simulink model "VehCtrlMdel240829_2018b"  (R2019b)
settings: Solver=FixedStepDiscrete  StartTime=0.0  StopTime=10.0  FixedStep=0.0005  RelTol=1e-3  EnableMultiTasking=on
values from neighbouring files (symbols this model uses):
  Ax_OffSet = 0.0    [VehCtrlMdelDictionary.sldd]
  Ay_OffSet = 0.0    [VehCtrlMdelDictionary.sldd]
  Caf = 460.0    [VehCtrlMdelDictionary.sldd]    (also in trqvparameter.m = 460)
  Car = 440.0    [VehCtrlMdelDictionary.sldd]    (also in trqvparameter.m = 440)
  dwf = 1.2    [VehCtrlMdelDictionary.sldd]    (also in trqvparameter.m)
  Iz = 105.0    [VehCtrlMdelDictionary.sldd]    (also in trqvparameter.m = 105)
  Ki = 1.0    [VehCtrlMdelDictionary.sldd]    (also in trqvparameter.m = 20)
  Kp = 2.0    [VehCtrlMdelDictionary.sldd]    (also in trqvparameter.m = 30)
  Ldwf = 1.2    [VehCtrlMdelDictionary.sldd]    (also in trqvparameter.m)
  Ldwr = 1.16    [VehCtrlMdelDictionary.sldd]    (also in trqvparameter.m)
  lf = 0.761    [VehCtrlMdelDictionary.sldd]    (also in trqvparameter.m)
  lr = 0.831    [VehCtrlMdelDictionary.sldd]    (also in trqvparameter.m)
  m = 340.0    [VehCtrlMdelDictionary.sldd]    (also in trqvparameter.m = 340)
  Offset_Angle = 0.0    [VehCtrlMdelDictionary.sldd]
  Qa = 0.1    [VehCtrlMdelDictionary.sldd]    (also in trqvparameter.m)
  Ra = 2.0    [VehCtrlMdelDictionary.sldd]    (also in trqvparameter.m = 2)
  RearRatio = 0.8    [VehCtrlMdelDictionary.sldd]
  Rt = 0.2    [VehCtrlMdelDictionary.sldd]    (also in trqvparameter.m)
  thr1 = 2.0    [VehCtrlMdelDictionary.sldd]    (also in trqvparameter.m = 2)
  thr2 = 0.5    [VehCtrlMdelDictionary.sldd]    (also in trqvparameter.m)
  thr3 = 0.8    [VehCtrlMdelDictionary.sldd]    (also in trqvparameter.m)
  thr4 = 0.5    [VehCtrlMdelDictionary.sldd]    (also in trqvparameter.m)
  thr5 = -0.5    [VehCtrlMdelDictionary.sldd]    (also in trqvparameter.m)
  TrqRquRate = 0.1    [VehCtrlMdelDictionary.sldd]    (also in trqvparameter.m)
  YawRate_OffSet = 0.0    [VehCtrlMdelDictionary.sldd]
undefined symbols (not defined in the file or in its folder): DiscIntNeverNeededParam, I_AN07_5V, I_AN08_5V, I_AN10_5V, I_SW01_L, I_SW02_L, I_SW03_L, O_SW12_HS1A, O_SW14_HS1A, PWM3
libraries: simulink x126, ec5744lib x77, canmsglib x18
(part 2 of 5)

== system VehCtrlMdel240829_2018b/OUTPUT/VCU2CLUSTER ==
  In1 : Inport
  TCS : Inport  Port=2
  function : TriggerPort  TriggerType=function-call  VariantControl=Variant
  Bus Selector : BusSelector  OutputSignals=signal2.APPBrk_BUS.Brk_F,signal2.MCU.MCU_state.Trq,signal2.APPBrk_BUS.Acc_POS,signal2.MCU.MCU_pwr.motor_temp,signal2.VehSpd_FLkph,signal2.MCU.MCU_state.Spd_R_kph,signal2.APPBrk_BUS.Brk_R,signal2.MCU.MCU_state.RPM
  Bus Selector1 : BusSelector  OutputSignals=TCS_TrqRequestFinal_Nm,TCS_flgActv
  CAN Pack : canmsglib/CAN Pack  CANdbFile=E:\candbc\cluster.dbc  MsgList=(none)  MsgName=New_Message_1  MsgIDType=Standard (11-bit identifier)  MsgIdentifier=291  MsgLength=8  Remote=off  ApplyMinMax=off  BusOutput=off  SignalInfo={'Brk_F','56','8','LE','signed','Standard','0','30','100','-3740','3910';'TCS_Trq_cmd','40','8','LE','unsigned','Standard','0','1','0','0','255';'TCS_flag','32','8','LE','signed','Standard','0','1','0','-Inf','Inf';'Trq_feedback','48','8','LE','signed','Standard','0','1','0','-128','250';'acc','24','8','LE','unsigned','Standard','0','1','0','0','100';'motor_temp','0','8','LE','unsigned','Standard','0','1','0','0','100';'veh_spd_F','8','8','LE','unsigned','Standard','0','1','0','0','120';'veh_spd_R','16','8','LE','unsigned','Standard','0','1','0','0','120'}
      settings: SourceProductName=Vehicle Network Toolbox  SourceProductBaseCode=VN  DataFormat=CANdb specified signals
  CAN Pack1 : canmsglib/CAN Pack  CANdbFile=E:\candbc\cluster.dbc  MsgList=(none)  MsgName=New_Message_2  MsgIDType=Standard (11-bit identifier)  MsgIdentifier=292  MsgLength=2  Remote=off  ApplyMinMax=off  BusOutput=off  SignalInfo={'Brk_R','0','8','LE','signed','Standard','0','30','100','-Inf','Inf';'RPM_feedback','8','8','LE','signed','Standard','0','1','0','-Inf','Inf'}
      settings: SourceProductName=Simulink Real-Time  SourceProductBaseCode=XP  DataFormat=CANdb specified signals
  CANPackMessage : ec5744lib/RapidECU_U3/04CANCommunication/CANPackMessage  datalength=8  sampletime=-1
      settings: SourceProductName=ECUCoder for MPC5744
  CANPackMessage1 : ec5744lib/HYFCU001/04CANCommunication/CANPackMessage  datalength=8  sampletime=-1
      settings: SourceProductName=ECUCoder for MPC5744
  CANTransmit : ec5744lib/RapidECU_U3/04CANCommunication/CANTransmit  canmodule=0  canbuffer=9  canmessageid=291  canmessagetype=Standard(11-bit ID)  datalength=8  sampletime=-1
      settings: SourceProductName=ECUCoder for MPC5744
  CANTransmit1 : ec5744lib/RapidECU_U3/04CANCommunication/CANTransmit  canmodule=0  canbuffer=10  canmessageid=292  canmessagetype=Standard(11-bit ID)  datalength=8  sampletime=-1
      settings: SourceProductName=ECUCoder for MPC5744
  Terminator1 : Terminator
  Terminator3 : Terminator
  wires:
  CANTransmit/1 -> Terminator3/1
  CANPackMessage/1 -> CANTransmit/1
  CAN Pack/1 -> CANPackMessage/1
  In1/1 -> Bus Selector/1
  Bus Selector/5 -> CAN Pack/7  "<VehSpd_FLkph>"
  Bus Selector/4 -> CAN Pack/6  "<motor_temp>"
  Bus Selector/3 -> CAN Pack/5  "<Acc_POS>"
  Bus Selector/6 -> CAN Pack/8  "<Spd_R_kph>"
  Bus Selector/1 -> CAN Pack/1  "<Brk_F>"
  Bus Selector/2 -> CAN Pack/4  "<Trq>"
  TCS/1 -> Bus Selector1/1
  Bus Selector1/2 -> CAN Pack/3  "<TCS_flgActv>"
  Bus Selector1/1 -> CAN Pack/2  "<TCS_TrqRequestFinal_Nm>"
  Bus Selector/7 -> CAN Pack1/1  "<Brk_R>"
  Bus Selector/8 -> CAN Pack1/2  "<RPM>"
  CAN Pack1/1 -> CANPackMessage1/1
  CANPackMessage1/1 -> CANTransmit1/1
  CANTransmit1/1 -> Terminator1/1

== system VehCtrlMdel240829_2018b/OUTPUT/VCU2EmraxMCU ==
  note: 0: 0Nm
      | 2: Trq mode
  note: 0: N
      | 2:D
  note: 加ramp
  note: 1.spd改成motor_rpm
      | 2.APP_bad改成acc_error
      | 3.设置模式的优先级
      | 4.车轮低负载（悬空），加最高车速限制
  In1 : Inport
  function : TriggerPort  TriggerType=function-call  VariantControl=(inherit)
  Bus Selector : BusSelector  OutputSignals=Trq_CUT,TrqR_cmd,VCU_SpdCmd_Emrax
  CAN Pack1 : canmsglib/CAN Pack  CANdbFile=E:\candbc\MCU_No1.dbc  MsgList=(none)  MsgName=VCU2MCU1_ID1  MsgIDType=Extended (29-bit identifier)  MsgIdentifier=146927393  MsgLength=8  Remote=off  ApplyMinMax=off  BusOutput=off  SignalInfo={'VCU2MCU_Control_mode_ID1','32','8','LE','unsigned','Standard','0','1','0','0','255';'VCU2MCU_Gear_ID1','40','2','LE','unsigned','Standard','0','1','0','0','3';'VCU2MCU_Speed_Limit_ID1','0','16','LE','unsigned','Standard','0','5.000000e-01','-10000','-10000','10000';'VCU2MCU_Torque_Control_ID1','16','16','LE','unsigned','Standard','0','1','0','0','1000'}
      settings: SourceProductName=Vehicle Network Toolbox  SourceProductBaseCode=VN  DataFormat=CANdb specified signals
  CANPackMessage : ec5744lib/RapidECU_U3/04CANCommunication/CANPackMessage  datalength=8  sampletime=-1
      settings: SourceProductName=ECUCoder for MPC5744
  CANTransmit : ec5744lib/RapidECU_U3/04CANCommunication/CANTransmit  canmodule=0  canbuffer=8  canmessageid=146927393  canmessagetype=Extended(29-bit ID)  datalength=8  sampletime=-1
      settings: SourceProductName=ECUCoder for MPC5744
  Cast To Boolean4 : DataTypeConversion  OutDataTypeStr=uint16
  Cast To Boolean6 : DataTypeConversion  OutDataTypeStr=uint16
  Constant13 : Constant  Value=2
  Constant17 : Constant  Value=0
  Constant19 : Constant  Value=2
  Constant20 : Constant  Value=0
  Data Type Conversion1 : DataTypeConversion  OutDataTypeStr=single
  Data Type Conversion2 : DataTypeConversion  OutDataTypeStr=int32
  MeaModule1 : ec5744lib/HYFCU001/07Calibration/MeaModule  signal=Gear_Trs
      settings: SourceProductName=ECUCoder for MPC5744
  MeaModule2 : ec5744lib/HYFCU001/07Calibration/MeaModule  signal=Mode_Trs
      settings: SourceProductName=ECUCoder for MPC5744
  Ramp : simulink/Sources/Ramp  Commented=on  slope=1  start=0  InitialOutput=0
  Switch2 : Switch  Criteria=u2 > Threshold
  Switch3 : Switch  Criteria=u2 > Threshold
  Terminator3 : Terminator
  wires:
  CANTransmit/1 -> Terminator3/1
  CAN Pack1/1 -> CANPackMessage/1
  CANPackMessage/1 -> CANTransmit/1
  MeaModule1/1 -> Cast To Boolean4/1
  Bus Selector/2 -> Data Type Conversion1/1  "<TrqR_cmd>"
  Constant20/1 -> Switch2/1
  Bus Selector/1 -> Switch2/2, Switch3/2  "<Trq_CUT>"
  Constant19/1 -> Switch2/3
  Constant13/1 -> Switch3/3
  Constant17/1 -> Switch3/1
  Switch3/1 -> MeaModule2/1
  Switch2/1 -> MeaModule1/1
  MeaModule2/1 -> Cast To Boolean6/1
  Data Type Conversion1/1 -> CAN Pack1/3
  Data Type Conversion2/1 -> CAN Pack1/4
  Cast To Boolean4/1 -> CAN Pack1/1
  Cast To Boolean6/1 -> CAN Pack1/2
  Bus Selector/3 -> Data Type Conversion2/1  "<VCU_SpdCmd_Emrax>"
  In1/1 -> Bus Selector/1

== system VehCtrlMdel240829_2018b/OUTPUT/WP_OUTPUT ==
  note: 数据类型转换
  aWaterPumpON : Inport
  LoadOfbWaterPump : Inport  Port=2
  function : TriggerPort  TriggerType=function-call  VariantControl=(inherit)
  Cast To Single : DataTypeConversion  OutDataTypeStr=boolean
  Cast To Single1 : DataTypeConversion  OutDataTypeStr=uint16
  Constant : Constant  Value=uint16(1000)  OutDataTypeStr=uint16  SampleTime=-1
  PowerDriverPWM : ec5744lib/RapidECU_U3/03PowerDriverPWM/PowerDriverPWM  channel=114:O_SW12_HS1A/PWM3  sampletime=-1
      settings: SourceProductName=ECUCoder for MPC5744
  PowerDriverSwitch(HS) : ec5744lib/RapidECU_U3/02PowerDriverSwitch/PowerDriverSwitch(HS)  channel=114:O_SW12_HS1A  sampletime=-1
      settings: SourceProductName=ECUCoder for MPC5744
  wires:
  LoadOfbWaterPump/1 -> Cast To Single1/1
  Constant/1 -> PowerDriverPWM/1
  aWaterPumpON/1 -> Cast To Single/1
  Cast To Single/1 -> PowerDriverSwitch(HS)/1
  Cast To Single1/1 -> PowerDriverPWM/2

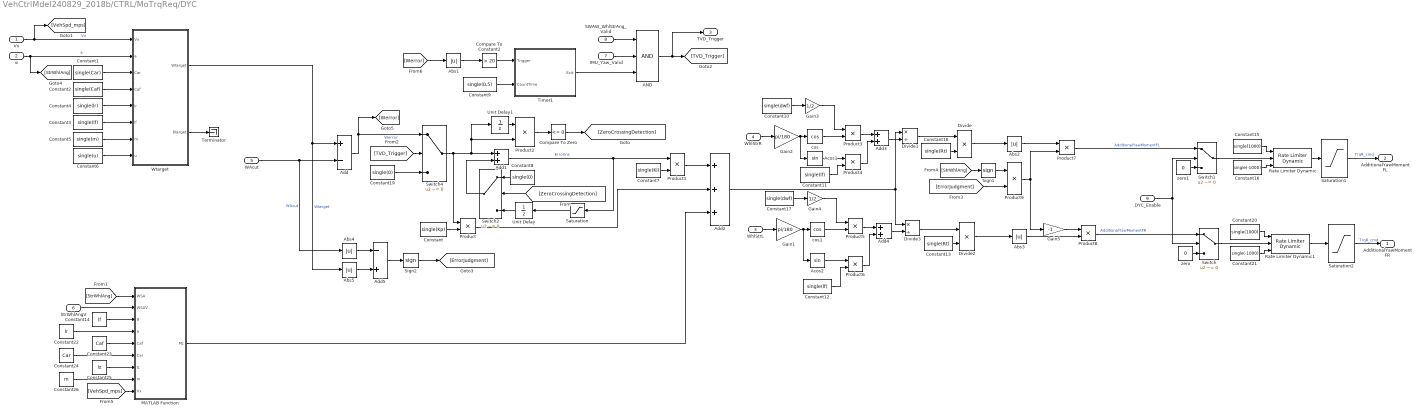
== system VehCtrlMdel240829_2018b/CTRL/MoTrqReq/DYC ==
  Vx : Inport
  α : Inport  Port=2
  WhlStrL : Inport  Port=3
  WhlStrR : Inport  Port=4
  WAcut : Inport  Port=5
  StrWhlAngV : Inport  Port=6
  IMU_Yaw_Valid : Inport  Port=7
  SWAW_WhlStrAng_Valid : Inport  Port=8
  "DYC_Enable " : Inport  Port=9
  AND : Logic  Inputs=3  AllPortsSameDT=off  OutDataTypeStr=boolean
  Abs{1..5} (5 alike) : Abs
  Acos1 : Trigonometry
  Acos2 : Trigonometry
  Add : Sum  Inputs=+-
  Add1 : Sum
  Add2 : Sum  Inputs=+++
  Add3 : Sum
  Add4 : Sum
  Add5 : Sum  Inputs=-+
  Compare To Constant2 : simulink/Logic and Bit Operations/Compare To Constant  relop=>  const=20  OutDataTypeStr=boolean
  Compare To Zero : simulink/Logic and Bit Operations/Compare To Zero  relop=<=  OutDataTypeStr=boolean
  Constant : Constant  Value=single(Kp)
  Constant1 : Constant  Value=single(Car)
  Constant10 : Constant  Value=single(dwf)
  Constant11 : Constant  Value=single(lf)
  Constant12 : Constant  Value=single(lf)
  Constant13 : Constant  Value=single(Rt)
  Constant14 : Constant  Value=lf
  Constant15 : Constant  Value=single(1000)
  Constant16 : Constant  Value=single(-1000)
  Constant17 : Constant  Value=single(dwf)
  Constant18 : Constant  Value=single(Rt)
  Constant19 : Constant  Value=single(0)
  Constant2 : Constant  Value=single(Caf)
  Constant20 : Constant  Value=single(1000)
  Constant21 : Constant  Value=single(-1000)
  Constant22 : Constant  Value=lr
  Constant23 : Constant  Value=Caf
  Constant24 : Constant  Value=Car
  Constant25 : Constant  Value=Iz
  Constant26 : Constant  Value=m
  Constant3 : Constant  Value=single(lf)
  Constant4 : Constant  Value=single(lr)
  Constant5 : Constant  Value=single(m)
  Constant6 : Constant  Value=single(u)
  Constant7 : Constant  Value=single(Ki)
  Constant8 : Constant  Value=single(0)
  Constant9 : Constant  Value=single(0.5)
  Divide : Product  Inputs=**
  Divide1 : Product  Inputs=*/
  Divide2 : Product  Inputs=**
  Divide3 : Product  Inputs=*/
  Gain1 : Gain  Gain=pi/180
  Gain2 : Gain  Gain=pi/180
  Gain3 : Gain  Gain=1/2
  Gain4 : Gain  Gain=1/2
  Gain5 : Gain  Gain=-1
  MATLAB Function : MATLAB Function  TreatAsAtomicUnit=on
  Product{,1..9} (10 alike) : Product
  Rate Limiter Dynamic : simulink/Discontinuities/Rate Limiter Dynamic
      settings: SourceProductName=Simulink
  Rate Limiter Dynamic1 : simulink/Discontinuities/Rate Limiter Dynamic
      settings: SourceProductName=Simulink
  Saturation : Saturate  UpperLimit=10  LowerLimit=-10
  Saturation1 : Saturate  UpperLimit=20  LowerLimit=-20
  Saturation2 : Saturate  UpperLimit=20  LowerLimit=-20
  Sign1 : Signum
  Sign2 : Signum
  Switch{,1..2,4} (4 alike) : Switch  Criteria=u2 ~= 0
  Terminator : Terminator
  Timer1 : Stateflow chart  TreatAsAtomicUnit=on
  Unit Delay : UnitDelay  SampleTime=-1  HasFrameUpgradeWarning=on
  Unit Delay1 : UnitDelay  SampleTime=-1  HasFrameUpgradeWarning=on
  Wtarget : MATLAB Function  TreatAsAtomicUnit=on
  cos : Trigonometry  Operator=cos
  cos1 : Trigonometry  Operator=cos
  zero : Constant  Value=0
  zero1 : Constant  Value=0
  AdditionalYawMomentFR : Outport  VectorParamsAs1DForOutWhenUnconnected=off
  AdditionalYawMomentFL : Outport  Port=2  VectorParamsAs1DForOutWhenUnconnected=off
  TVD_Trigger : Outport  Port=3  VectorParamsAs1DForOutWhenUnconnected=off
  wires:
  Constant2/1 -> Wtarget/4(Caf)
  Wtarget/1(Wtarget) -> Add/1, Abs5/1  "Wtarget"
  Vx/1 -> [VehSpd_mps], Wtarget/1(Vx)  "Vx"
  Constant6/1 -> Wtarget/8(u)
  Constant5/1 -> Wtarget/7(m)
  Constant1/1 -> Wtarget/3(Car)
  Constant3/1 -> Wtarget/6(lf)
  α/1 -> [StrWhlAng], Wtarget/2(a)  "a"
  Constant4/1 -> Wtarget/5(lr)
  Product8/1 -> Switch/1  "AdditionalYawMomentFR"
  Product7/1 -> Switch1/1  "AdditionalYawMomentFL"
  Wtarget/2(btarget) -> Terminator/1
  Switch/1 -> Rate Limiter Dynamic1/2
  Switch1/1 -> Rate Limiter Dynamic/2
  "DYC_Enable "/1 -> Switch1/2, Switch/2
  zero/1 -> Switch/3
  zero1/1 -> Switch1/3
  Compare To Zero/1 -> [ZeroCrossingDetection]
  Abs3/1 -> Product8/2
  Abs5/1 -> Add5/2
  Abs4/1 -> Add5/1
  Constant19/1 -> Switch4/3
  Add5/1 -> Sign2/1
  Constant12/1 -> Product6/2
  Sign2/1 -> [ErrorJudgment]
  Saturation/1 -> Unit Delay/1
  Divide/1 -> Abs2/1
  [ErrorJudgment] -> Product9/2
  Unit Delay/1 -> Switch2/3
  Add1/1 -> Saturation/1, Product1/1  "ErrorIns"
  Add3/1 -> Divide1/2
  Gain5/1 -> Product8/1
  Product4/1 -> Add3/2
  Abs2/1 -> Product7/1
  Acos2/1 -> Product6/1
  Add/1 -> [Werror], Switch4/1  "Werror"
  Gain1/1 -> cos1/1, Acos2/1
  Constant15/1 -> Rate Limiter Dynamic/1
  Divide1/1 -> Divide/1
  WhlStrL/1 -> Gain1/1
  cos/1 -> Product3/2
  [TVD_Trigger] -> Switch4/2
  Constant11/1 -> Product4/2
  Product5/1 -> Add4/1
  Product3/1 -> Add3/1
  Constant10/1 -> Gain3/1
  Gain2/1 -> Acos1/1, cos/1
  Gain3/1 -> Product3/1
  Constant8/1 -> Switch2/1
  Product6/1 -> Add4/2
  Acos1/1 -> Product4/1
  WhlStrR/1 -> Gain2/1
  Add4/1 -> Divide3/2
  Constant18/1 -> Divide/2
  Constant17/1 -> Gain4/1
  Switch4/1 -> Add1/1, Unit Delay1/1, Product2/2, Product/1
  WAcut/1 -> Add/2, Abs4/1  "WAcut"
  Product/1 -> Add2/2
  Abs1/1 -> Compare To Constant2/1
  [ZeroCrossingDetection] -> Switch2/2
  Compare To Constant2/1 -> Timer1/1(Trigger)
  Divide3/1 -> Divide2/1
  Gain4/1 -> Product5/1
  Constant13/1 -> Divide2/2
  Switch2/1 -> Add1/2
  Product9/1 -> Gain5/1, Product7/2
  cos1/1 -> Product5/2
  Constant16/1 -> Rate Limiter Dynamic/3
  Sign1/1 -> Product9/1
  Divide2/1 -> Abs3/1
  Constant/1 -> Product/2
  Constant7/1 -> Product1/2
  Product1/1 -> Add2/1
  Rate Limiter Dynamic/1 -> Saturation1/1
  Constant21/1 -> Rate Limiter Dynamic1/3
  Constant20/1 -> Rate Limiter Dynamic1/1
  Rate Limiter Dynamic1/1 -> Saturation2/1
  Add2/1 -> Divide3/1, Divide1/1
  Saturation1/1 -> AdditionalYawMomentFL/1  "TrqR_cmd"
  Saturation2/1 -> AdditionalYawMomentFR/1  "TrqR_cmd"
  [StrWhlAng] -> Sign1/1
  StrWhlAngV/1 -> MATLAB Function/2(WSAV)
  Constant9/1 -> Timer1/2(CountTime)
  Timer1/1(Exit) -> AND/3
  IMU_Yaw_Valid/1 -> AND/2
  SWAW_WhlStrAng_Valid/1 -> AND/1
  AND/1 -> TVD_Trigger/1, [TVD_Trigger]
  MATLAB Function/1(Mz) -> Add2/3
  [StrWhlAng] -> MATLAB Function/1(WSA)
  Constant14/1 -> MATLAB Function/3(lf)
  Constant22/1 -> MATLAB Function/4(lr)
  Constant23/1 -> MATLAB Function/5(Caf)
  Constant24/1 -> MATLAB Function/6(Car)
  Constant25/1 -> MATLAB Function/7(Iz)
  Constant26/1 -> MATLAB Function/8(m)
  [VehSpd_mps] -> MATLAB Function/9(Vx)
  Unit Delay1/1 -> Product2/1
  Product2/1 -> Compare To Zero/1
  [Werror] -> Abs1/1

== system VehCtrlMdel240829_2018b/CTRL/MoTrqReq/Subsystem ==
  SingleAMKPowerLimit_KW : Inport
  SingleEmraxPowerLimit_KW : Inport  Port=2
  MCFL_ActualVelocity : Inport  Port=3
  MCFR_ActualVelocity : Inport  Port=4
  RPM : Inport  Port=5
  Add : Sum  Inputs=+-
  Add1 : Sum
  Add2 : Sum
  Add3 : Sum
  Add4 : Sum  Inputs=+-
  Constant : Constant
  Constant1 : Constant  Value=single(9550)  OutDataTypeStr=single
  Constant2 : Constant  Value=single(9550)  OutDataTypeStr=single
  Constant3 : Constant
  Constant5 : Constant  Value=single(9550)  OutDataTypeStr=single
  Divide : Product  Inputs=*/
  Divide1 : Product  Inputs=*/
  Divide2 : Product  Inputs=*/
  Max : MinMax  Function=max  Inputs=2
  Max1 : MinMax  Function=max  Inputs=2
  Max2 : MinMax  Function=max  Inputs=2
  MaxPwr : Constant  Value=single(63)  OutDataTypeStr=single
  MaxPwr1 : Constant  Value=single(7)  OutDataTypeStr=single
  MaxPwr2 : Constant  Value=single(7)  OutDataTypeStr=single
  Product{,1..5} (6 alike) : Product
  RPM_min : Constant  Value=single(10)  OutDataTypeStr=single
  RPM_min1 : Constant  Value=single(1)  OutDataTypeStr=single
  RPM_min2 : Constant  Value=single(10)  OutDataTypeStr=single
  RPM_min3 : Constant  Value=single(1)  OutDataTypeStr=single
  RPM_min4 : Constant  Value=single(10)  OutDataTypeStr=single
  RPM_min5 : Constant  Value=single(1)  OutDataTypeStr=single
  TrqLimEmrax_Nm : Outport
  TrqLimFR_Nm : Outport  Port=2
  TrqLimFL_Nm : Outport  Port=3
  wires:
  Max/1 -> Divide/2
  Divide/1 -> TrqLimEmrax_Nm/1  "TrqLim_Nm"
  RPM_min1/1 -> Max/2
  Constant5/1 -> Product/2
  RPM/1 -> Add1/1
  Product/1 -> Divide/1
  RPM_min/1 -> Add1/2
  Add1/1 -> Max/1
  Add2/1 -> Max1/1
  RPM_min2/1 -> Add2/2
  MaxPwr1/1 -> Product4/1
  Product1/1 -> Divide1/1
  MCFR_ActualVelocity/1 -> Add2/1
  Constant1/1 -> Product1/2
  RPM_min3/1 -> Max1/2
  Divide1/1 -> TrqLimFR_Nm/1  "TrqLim_Nm"
  Max1/1 -> Divide1/2
  Max2/1 -> Divide2/2
  Divide2/1 -> TrqLimFL_Nm/1  "TrqLim_Nm"
  RPM_min5/1 -> Max2/2
  Constant2/1 -> Product2/2
  MCFL_ActualVelocity/1 -> Add3/1
  Product2/1 -> Divide2/1
  RPM_min4/1 -> Add3/2
  Add3/1 -> Max2/1
  MaxPwr/1 -> Product5/1
  Add/1 -> Product5/2
  Product5/1 -> Product/1
  Product3/1 -> Product2/1
  Add4/1 -> Product3/2, Product4/2
  Product4/1 -> Product1/1
  Constant/1 -> Add4/1
  MaxPwr2/1 -> Product3/1
  SingleAMKPowerLimit_KW/1 -> Add4/2
  SingleEmraxPowerLimit_KW/1 -> Add/2
  Constant3/1 -> Add/1

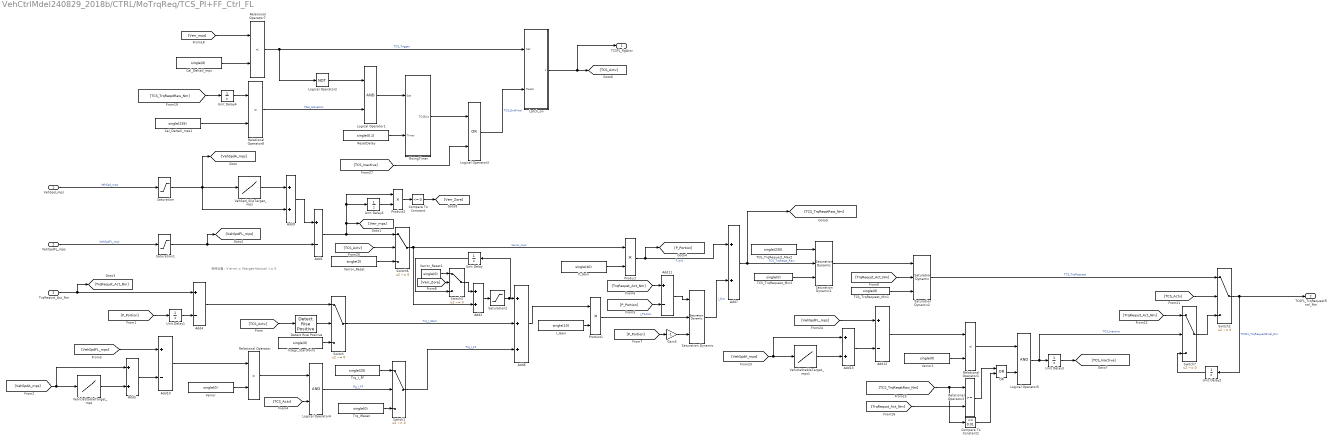
== system VehCtrlMdel240829_2018b/CTRL/MoTrqReq/TCS_PI+FF_Ctrl_FL ==
  note: 特殊设置：V error = Vtarget-Vactual <= 0
  VehSpd_mps : Inport
  VehSpdFL_mps : Inport  Port=2
  TrqRequst_Act_Nm : Inport  Port=3
  Add{1,4,10..12} (5 alike) : Sum  Inputs=+-
  Add{2,5,7,9,13} (5 alike) : Sum
  Add6 : Sum  Inputs=+++
  Cal_DeltaV_mps : Constant  Value=single(0)
  Cal_DeltaV_mps1 : Constant  Value=single(235)
  Compare To Constant : simulink/Logic and Bit Operations/Compare To Constant  relop=<=  const=0  OutDataTypeStr=boolean
  Compare To Constant2 : simulink/Logic and Bit Operations/Compare To Constant  relop=<=  const=0.01  OutDataTypeStr=boolean
  Detect Rise Positive : simulink/Logic and Bit Operations/Detect Rise Positive  vinit=0  OutDataTypeStr=boolean
  Gain3 : Gain  Gain=-1
  I_Gain : Constant  Value=single(10)
  Integr_StartPoint : Constant  Value=single(0)
  Latch_on : Subsystem
  Logical Operator1 : Logic  AllPortsSameDT=off  OutDataTypeStr=boolean
  Logical Operator2 : Logic  Operator=NOT  AllPortsSameDT=off  OutDataTypeStr=boolean
  Logical Operator3 : Logic  Operator=OR  AllPortsSameDT=off  OutDataTypeStr=boolean
  Logical Operator4 : Logic  AllPortsSameDT=off  OutDataTypeStr=boolean
  Logical Operator5 : Logic  AllPortsSameDT=off  OutDataTypeStr=boolean
  OR : Logic  Operator=OR  AllPortsSameDT=off  OutDataTypeStr=boolean
  P_Gain : Constant  Value=single(40)
  Product : Product
  Product1 : Product
  Product2 : Product
  Relational Operator : RelationalOperator  Operator=<  OutDataTypeStr=boolean  RndMeth=Simplest
  Relational Operator1 : RelationalOperator  Operator=<  OutDataTypeStr=boolean  RndMeth=Simplest
  Relational Operator2 : RelationalOperator  OutDataTypeStr=boolean  RndMeth=Simplest
  Relational Operator7 : RelationalOperator  Operator=<  OutDataTypeStr=boolean  RndMeth=Simplest
  Relational Operator8 : RelationalOperator  Operator=>  OutDataTypeStr=boolean  RndMeth=Simplest
  ResetDelay : Constant  Value=single(0.1)
  RisingTimer : Subsystem
  Saturation : Saturate  UpperLimit=40  LowerLimit=0
  Saturation Dynamic : simulink/Discontinuities/Saturation Dynamic  OutMin=[]  OutMax=[]  OutDataTypeStr=Inherit: Same as second input  OutDataType=fixdt(1, 16)  OutScaling=2^-10  DoSatur=off
  Saturation Dynamic1 : simulink/Discontinuities/Saturation Dynamic  OutMin=[]  OutMax=[]  OutDataTypeStr=Inherit: Same as second input  OutDataType=fixdt(1, 16)  OutScaling=2^-10  DoSatur=off
  Saturation Dynamic2 : simulink/Discontinuities/Saturation Dynamic  OutMin=[]  OutMax=[]  OutDataTypeStr=Inherit: Same as second input  OutDataType=fixdt(1, 16)  OutScaling=2^-10  DoSatur=off
  Saturation1 : Saturate  UpperLimit=50  LowerLimit=0
  Saturation2 : Saturate  UpperLimit=400  LowerLimit=-100
  Switch{,1..3,6..7} (6 alike) : Switch  Criteria=u2 ~= 0
  TCS_TrqRequest_Max2 : Constant  Value=single(235)
  TCS_TrqRequest_Min1 : Constant  Value=single(0)
  TCS_TrqRequest_Min2 : Constant  Value=single(0)
  Trq_IReset : Constant  Value=single(0)
  Trq_I_FF : Constant  Value=single(20)
  Unit Delay{,1..5} (6 alike) : UnitDelay  SampleTime=-1  HasFrameUpgradeWarning=on
  VehSpd_SlipTarget_mps : Lookup_n-D  NumberOfTableDimensions=1  BreakpointsForDimension1=[0,3,25,30]  Table=[0.3,0.3,2.5,2.5]  ExtrapMethod=Clip  InternalRulePriority=Speed  RndMeth=Simplest  InputSameDT=on
  VehicleStableTarget_mps : Lookup_n-D  NumberOfTableDimensions=1  BreakpointsForDimension1=[0,3,25,30]  Table=[0.4,0.4,1.2,1.2]  ExtrapMethod=Clip  InternalRulePriority=Speed  RndMeth=Simplest  InputSameDT=on
  VehicleStableTarget_mps1 : Lookup_n-D  NumberOfTableDimensions=1  BreakpointsForDimension1=[0,3,25,30]  Table=[0.4,0.4,1.2,1.2]  ExtrapMethod=Clip  InternalRulePriority=Speed  RndMeth=Simplest  InputSameDT=on
  Verror : Constant  Value=single(0)
  Verror1 : Constant  Value=single(0)
  Verror_Reset : Constant  Value=single(0)
  Verror_Reset1 : Constant  Value=single(0)
  TCSFL_flgActv : Outport
  TCSFL_TrqRequestFinal_Nm : Outport  Port=2
  wires:
  Switch2/1 -> TCSFL_TrqRequestFinal_Nm/1, Unit Delay2/1  "TCSFL_TrqRequestFinal_Nm"
  Saturation/1 -> Add9/2, VehSpd_SlipTarget_mps/1, [VehSpdA_mps]
  Gain3/1 -> Saturation Dynamic/3
  [P_Portion] -> Gain3/1
  P_Gain/1 -> Product/2
  Unit Delay/1 -> Switch3/3
  Add2/1 -> Saturation2/1
  [TrqRequst_Act_Nm] -> Add11/1
  Saturation2/1 -> Unit Delay/1, Add6/1
  Switch/1 -> Add6/2  "Trq_I_Start"
  Saturation Dynamic/1 -> Add7/2  "I_Out"
  VehSpd_mps/1 -> Saturation/1  "VehSpd_mps"
  Saturation1/1 -> Add1/2, [VehSpdFL_mps]
  Product1/1 -> Saturation Dynamic/2  "I_Portion"
  TrqRequst_Act_Nm/1 -> Add4/1, [TrqRequst_Act_Nm]
  Add6/1 -> Product1/1
  TCS_TrqRequest_Min1/1 -> Saturation Dynamic2/3
  Detect Rise Positive/1 -> Switch/2
  Integr_StartPoint/1 -> Switch/3
  I_Gain/1 -> Product1/2
  Saturation Dynamic2/1 -> Switch2/1  "TCS_TrqRequest"
  Add7/1 -> Saturation Dynamic1/2, [TCS_TrqReqstRaw_Nm]  "TCS_TrqReqst_Raw"
  [TrqRequst_Act_Nm] -> Saturation Dynamic2/2
  VehSpd_SlipTarget_mps/1 -> Add9/1
  Add9/1 -> Add1/1
  [Verr_mps] -> Relational Operator7/1
  Cal_DeltaV_mps/1 -> Relational Operator7/2
  Relational Operator7/1 -> Latch_on/1(Set), Logical Operator2/1  "TCS_Trigger"
  [TCS_TrqReqstRaw_Nm] -> Unit Delay4/1
  Logical Operator2/1 -> Logical Operator1/1
  Relational Operator8/1 -> Logical Operator1/2  "fSat_Actuators"
  Cal_DeltaV_mps1/1 -> Relational Operator8/2
  Logical Operator1/1 -> RisingTimer/1(Set)
  ResetDelay/1 -> RisingTimer/2(Timer)
  RisingTimer/1(TCSExit) -> Logical Operator3/1
  Logical Operator3/1 -> Latch_on/2(Reset)  "TCS_ExitFinal"
  Latch_on/1(flg_TCSActv) -> TCSFL_flgActv/1, [TCS_Actv]
  [TCS_Actv] -> Switch6/2
  Verror_Reset/1 -> Switch6/3
  Switch6/1 -> Product/1, Add2/2  "Verror_mps"
  Product/1 -> [P_Portion], Add7/1  "P_out"
  [TCS_Actv] -> Detect Rise Positive/1
  [P_Portion] -> Unit Delay1/1
  Add4/1 -> Switch/1
  Unit Delay1/1 -> Add4/2
  [VehSpdA_mps] -> Add5/1, VehicleStableTarget_mps/1
  VehicleStableTarget_mps/1 -> Add5/2
  Add5/1 -> Add10/2
  [VehSpdFL_mps] -> Add10/1
  Add10/1 -> Relational Operator/1
  Verror/1 -> Relational Operator/2
  Relational Operator/1 -> Logical Operator4/1
  [TCS_Actv] -> Logical Operator4/2
  Logical Operator4/1 -> Switch1/2  "flg_I_FF"
  Trq_I_FF/1 -> Switch1/1
  Trq_IReset/1 -> Switch1/3
  Switch1/1 -> Add6/3  "Trq_I_FF"
  [P_Portion] -> Add11/2
  Add11/1 -> Saturation Dynamic/1
  [TCS_Actv] -> Switch2/2
  Switch7/1 -> Switch2/3
  [TrqRequst_Act_Nm] -> Switch7/1
  Verror1/1 -> Relational Operator1/2
  Add12/1 -> Relational Operator1/1
  [VehSpdFL_mps] -> Add12/1
  Add13/1 -> Add12/2
  VehicleStableTarget_mps1/1 -> Add13/2
  [VehSpdA_mps] -> VehicleStableTarget_mps1/1, Add13/1
  [TCS_TrqReqstRaw_Nm] -> Compare To Constant2/1, Relational Operator2/1
  [TrqRequst_Act_Nm] -> Relational Operator2/2
  Relational Operator1/1 -> Logical Operator5/1
  Logical Operator5/1 -> Switch7/2, Unit Delay3/1  "TCS_Inactive"
  Unit Delay3/1 -> [TCS_Inactive]
  [TCS_Inactive] -> Logical Operator3/2
  Unit Delay4/1 -> Relational Operator8/1
  VehSpdFL_mps/1 -> Saturation1/1  "VehSpdFL_mps"
  Saturation Dynamic1/1 -> Saturation Dynamic2/1
  TCS_TrqRequest_Max2/1 -> Saturation Dynamic1/1
  TCS_TrqRequest_Min2/1 -> Saturation Dynamic1/3
  Switch3/1 -> Add2/1
  Verror_Reset1/1 -> Switch3/1
  [Verr_Zore] -> Switch3/2
  Product2/1 -> Compare To Constant/1
  Unit Delay5/1 -> Product2/2
  Add1/1 -> Switch6/1, [Verr_mps], Unit Delay5/1, Product2/1
  Compare To Constant/1 -> [Verr_Zore]
  Unit Delay2/1 -> Switch7/3
  Compare To Constant2/1 -> OR/2
  Relational Operator2/1 -> OR/1
  OR/1 -> Logical Operator5/2

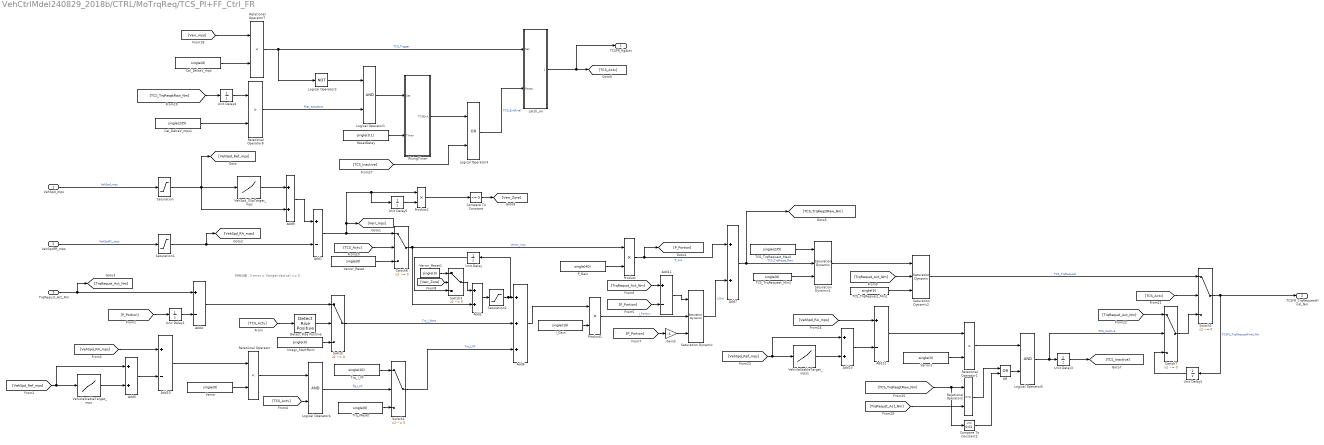
== system VehCtrlMdel240829_2018b/CTRL/MoTrqReq/TCS_PI+FF_Ctrl_FR ==
  note: 特殊设置：V error = Vtarget-Vactual <= 0
  VehSpd_mps : Inport
  VehSpdFR_mps : Inport  Port=2
  TrqRequst_Act_Nm : Inport  Port=3
  Add{1,4,10..12} (5 alike) : Sum  Inputs=+-
  Add{2,5,7,9,13} (5 alike) : Sum
  Add6 : Sum  Inputs=+++
  Cal_DeltaV_mps : Constant  Value=single(0)
  Cal_DeltaV_mps1 : Constant  Value=single(235)
  Compare To Constant : simulink/Logic and Bit Operations/Compare To Constant  relop=<=  const=0  OutDataTypeStr=boolean
  Compare To Constant2 : simulink/Logic and Bit Operations/Compare To Constant  relop=<=  const=0.01  OutDataTypeStr=boolean
  Detect Rise Positive : simulink/Logic and Bit Operations/Detect Rise Positive  vinit=0  OutDataTypeStr=boolean
  Gain3 : Gain  Gain=-1
  I_Gain : Constant  Value=single(10)
  Integr_StartPoint : Constant  Value=single(0)
  Latch_on : Subsystem
  Logical Operator1 : Logic  AllPortsSameDT=off  OutDataTypeStr=boolean
  Logical Operator2 : Logic  Operator=NOT  AllPortsSameDT=off  OutDataTypeStr=boolean
  Logical Operator3 : Logic  Operator=OR  AllPortsSameDT=off  OutDataTypeStr=boolean
  Logical Operator4 : Logic  AllPortsSameDT=off  OutDataTypeStr=boolean
  Logical Operator5 : Logic  AllPortsSameDT=off  OutDataTypeStr=boolean
  OR : Logic  Operator=OR  AllPortsSameDT=off  OutDataTypeStr=boolean
  P_Gain : Constant  Value=single(40)
  Product : Product
  Product1 : Product
  Product2 : Product
  Relational Operator : RelationalOperator  Operator=<  OutDataTypeStr=boolean  RndMeth=Simplest
  Relational Operator1 : RelationalOperator  Operator=<  OutDataTypeStr=boolean  RndMeth=Simplest
  Relational Operator2 : RelationalOperator  OutDataTypeStr=boolean  RndMeth=Simplest
  Relational Operator7 : RelationalOperator  Operator=<  OutDataTypeStr=boolean  RndMeth=Simplest
  Relational Operator8 : RelationalOperator  Operator=>  OutDataTypeStr=boolean  RndMeth=Simplest
  ResetDelay : Constant  Value=single(0.1)
  RisingTimer : Subsystem
  Saturation : Saturate  UpperLimit=40  LowerLimit=0
  Saturation Dynamic : simulink/Discontinuities/Saturation Dynamic  OutMin=[]  OutMax=[]  OutDataTypeStr=Inherit: Same as second input  OutDataType=fixdt(1, 16)  OutScaling=2^-10  DoSatur=off
  Saturation Dynamic1 : simulink/Discontinuities/Saturation Dynamic  OutMin=[]  OutMax=[]  OutDataTypeStr=Inherit: Same as second input  OutDataType=fixdt(1, 16)  OutScaling=2^-10  DoSatur=off
  Saturation Dynamic2 : simulink/Discontinuities/Saturation Dynamic  OutMin=[]  OutMax=[]  OutDataTypeStr=Inherit: Same as second input  OutDataType=fixdt(1, 16)  OutScaling=2^-10  DoSatur=off
  Saturation1 : Saturate  UpperLimit=50  LowerLimit=0
  Saturation2 : Saturate  UpperLimit=400  LowerLimit=-100
  Switch{,1..3,6..7} (6 alike) : Switch  Criteria=u2 ~= 0
  TCS_TrqRequest_Max2 : Constant  Value=single(235)
  TCS_TrqRequest_Min1 : Constant  Value=single(0)
  TCS_TrqRequest_Min2 : Constant  Value=single(0)
  Trq_IReset : Constant  Value=single(0)
  Trq_I_FF : Constant  Value=single(20)
  Unit Delay{,1..5} (6 alike) : UnitDelay  SampleTime=-1  HasFrameUpgradeWarning=on
  VehSpd_SlipTarget_mps : Lookup_n-D  NumberOfTableDimensions=1  BreakpointsForDimension1=[0,3,25,30]  Table=[0.3,0.3,2.5,2.5]  ExtrapMethod=Clip  InternalRulePriority=Speed  RndMeth=Simplest  InputSameDT=on
  VehicleStableTarget_mps : Lookup_n-D  NumberOfTableDimensions=1  BreakpointsForDimension1=[0,3,25,30]  Table=[0.4,0.4,1.2,1.2]  ExtrapMethod=Clip  InternalRulePriority=Speed  RndMeth=Simplest  InputSameDT=on
  VehicleStableTarget_mps1 : Lookup_n-D  NumberOfTableDimensions=1  BreakpointsForDimension1=[0,3,25,30]  Table=[0.4,0.4,1.2,1.2]  ExtrapMethod=Clip  InternalRulePriority=Speed  RndMeth=Simplest  InputSameDT=on
  Verror : Constant  Value=single(0)
  Verror1 : Constant  Value=single(0)
  Verror_Reset : Constant  Value=single(0)
  Verror_Reset1 : Constant  Value=single(0)
  TCSFR_flgActv : Outport
  TCSFR_TrqRequestFinal_Nm : Outport  Port=2
  wires:
  [Verr_Zore] -> Switch3/2
  Verror_Reset1/1 -> Switch3/1
  Switch3/1 -> Add2/1
  TCS_TrqRequest_Min2/1 -> Saturation Dynamic1/3
  TCS_TrqRequest_Max2/1 -> Saturation Dynamic1/1
  Saturation Dynamic1/1 -> Saturation Dynamic2/1
  VehSpdFR_mps/1 -> Saturation1/1  "VehSpdFL_mps"
  Unit Delay4/1 -> Relational Operator8/1
  [TCS_Inactive] -> Logical Operator3/2
  Unit Delay3/1 -> [TCS_Inactive]
  Logical Operator5/1 -> Switch7/2, Unit Delay3/1  "TCS_Inactive"
  Relational Operator1/1 -> Logical Operator5/1
  [TrqRequst_Act_Nm] -> Relational Operator2/2
  [TCS_TrqReqstRaw_Nm] -> Compare To Constant2/1, Relational Operator2/1
  [VehSpd_Ref_mps] -> Add13/1, VehicleStableTarget_mps1/1
  VehicleStableTarget_mps1/1 -> Add13/2
  Add13/1 -> Add12/2
  [VehSpd_RA_mps] -> Add12/1
  Add12/1 -> Relational Operator1/1
  Verror1/1 -> Relational Operator1/2
  [TrqRequst_Act_Nm] -> Switch7/1
  Switch7/1 -> Switch2/3
  [TCS_Actv] -> Switch2/2
  Add11/1 -> Saturation Dynamic/1
  [P_Portion] -> Add11/2
  Switch1/1 -> Add6/3  "Trq_I_FF"
  Trq_IReset/1 -> Switch1/3
  Trq_I_FF/1 -> Switch1/1
  Logical Operator4/1 -> Switch1/2  "flg_I_FF"
  [TCS_Actv] -> Logical Operator4/2
  Relational Operator/1 -> Logical Operator4/1
  Verror/1 -> Relational Operator/2
  Add10/1 -> Relational Operator/1
  [VehSpd_RA_mps] -> Add10/1
  Add5/1 -> Add10/2
  VehicleStableTarget_mps/1 -> Add5/2
  [VehSpd_Ref_mps] -> VehicleStableTarget_mps/1, Add5/1
  Unit Delay1/1 -> Add4/2
  Add4/1 -> Switch/1
  [P_Portion] -> Unit Delay1/1
  [TCS_Actv] -> Detect Rise Positive/1
  Product/1 -> Add7/1, [P_Portion]  "P_out"
  Switch6/1 -> Add2/2, Product/1  "Verror_mps"
  Verror_Reset/1 -> Switch6/3
  [TCS_Actv] -> Switch6/2
  Latch_on/1(flg_TCSActv) -> [TCS_Actv], TCSFR_flgActv/1
  Logical Operator3/1 -> Latch_on/2(Reset)  "TCS_ExitFinal"
  RisingTimer/1(TCSExit) -> Logical Operator3/1
  ResetDelay/1 -> RisingTimer/2(Timer)
  Logical Operator1/1 -> RisingTimer/1(Set)
  Cal_DeltaV_mps1/1 -> Relational Operator8/2
  Relational Operator8/1 -> Logical Operator1/2  "fSat_Actuators"
  Logical Operator2/1 -> Logical Operator1/1
  [TCS_TrqReqstRaw_Nm] -> Unit Delay4/1
  Relational Operator7/1 -> Logical Operator2/1, Latch_on/1(Set)  "TCS_Trigger"
  Cal_DeltaV_mps/1 -> Relational Operator7/2
  [Verr_mps] -> Relational Operator7/1
  Add9/1 -> Add1/1
  VehSpd_SlipTarget_mps/1 -> Add9/1
  [TrqRequst_Act_Nm] -> Saturation Dynamic2/2
  Add7/1 -> [TCS_TrqReqstRaw_Nm], Saturation Dynamic1/2  "TCS_TrqReqst_Raw"
  Saturation Dynamic2/1 -> Switch2/1  "TCS_TrqRequest"
  I_Gain/1 -> Product1/2
  Integr_StartPoint/1 -> Switch/3
  Detect Rise Positive/1 -> Switch/2
  TCS_TrqRequest_Min1/1 -> Saturation Dynamic2/3
  Add6/1 -> Product1/1
  TrqRequst_Act_Nm/1 -> [TrqRequst_Act_Nm], Add4/1
  Product1/1 -> Saturation Dynamic/2  "I_Portion"
  Saturation1/1 -> [VehSpd_RA_mps], Add1/2
  VehSpd_mps/1 -> Saturation/1  "VehSpd_mps"
  Saturation Dynamic/1 -> Add7/2  "I_Out"
  Switch/1 -> Add6/2  "Trq_I_Start"
  Saturation2/1 -> Add6/1, Unit Delay/1
  [TrqRequst_Act_Nm] -> Add11/1
  Add2/1 -> Saturation2/1
  Unit Delay/1 -> Switch3/3
  P_Gain/1 -> Product/2
  [P_Portion] -> Gain3/1
  Gain3/1 -> Saturation Dynamic/3
  Saturation/1 -> [VehSpd_Ref_mps], VehSpd_SlipTarget_mps/1, Add9/2
  Switch2/1 -> Unit Delay2/1, TCSFR_TrqRequestFinal_Nm/1  "TCSFL_TrqRequestFinal_Nm"
  Product2/1 -> Compare To Constant/1
  Unit Delay5/1 -> Product2/2
  Add1/1 -> Unit Delay5/1, Product2/1, [Verr_mps], Switch6/1
  Compare To Constant/1 -> [Verr_Zore]
  Unit Delay2/1 -> Switch7/3
  Compare To Constant2/1 -> OR/2
  Relational Operator2/1 -> OR/1
  OR/1 -> Logical Operator5/2

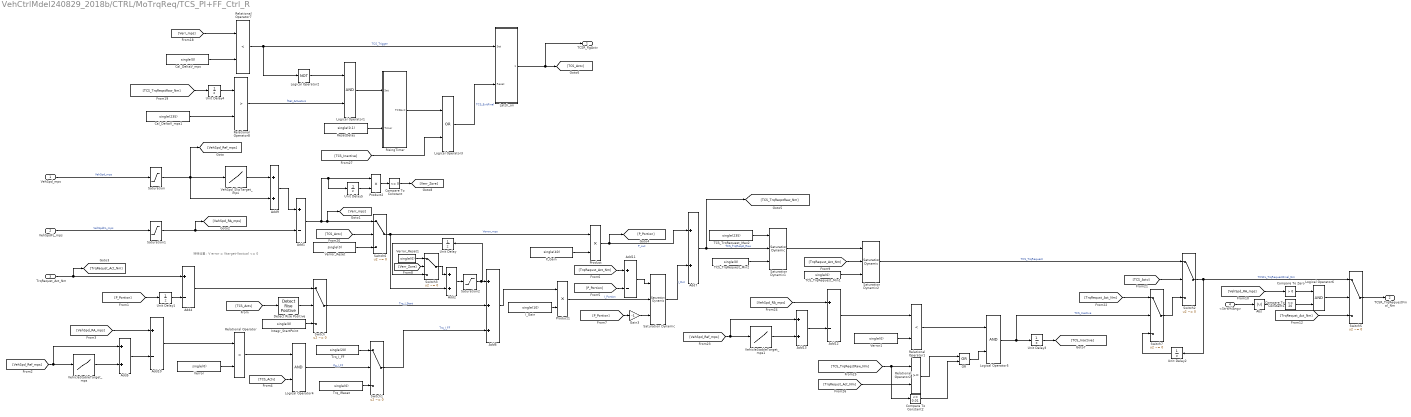
== system VehCtrlMdel240829_2018b/CTRL/MoTrqReq/TCS_PI+FF_Ctrl_R ==
  note: 特殊设置：V error = Vtarget-Vactual <= 0
  VehSpd_mps : Inport
  VehSpdFL_mps : Inport  Port=2
  TrqRequst_Act_Nm : Inport  Port=3
  <StrWhlAng> : Inport  Port=4
  Abs : Abs
  Add{1,4,10..12} (5 alike) : Sum  Inputs=+-
  Add{2,5,7,9,13} (5 alike) : Sum
  Add6 : Sum  Inputs=+++
  Cal_DeltaV_mps : Constant  Value=single(0)
  Cal_DeltaV_mps1 : Constant  Value=single(235)
  Compare To Constant : simulink/Logic and Bit Operations/Compare To Constant  relop=<=  const=0  OutDataTypeStr=boolean
  Compare To Constant1 : simulink/Logic and Bit Operations/Compare To Constant  relop=<=  const=20  OutDataTypeStr=boolean
  Compare To Constant2 : simulink/Logic and Bit Operations/Compare To Constant  relop=<=  const=0.01  OutDataTypeStr=boolean
  Compare To Zero : simulink/Logic and Bit Operations/Compare To Zero  relop=>  OutDataTypeStr=boolean
  Detect Rise Positive : simulink/Logic and Bit Operations/Detect Rise Positive  vinit=0  OutDataTypeStr=boolean
  Gain3 : Gain  Gain=-1
  I_Gain : Constant  Value=single(10)
  Integr_StartPoint : Constant  Value=single(0)
  Latch_on : Subsystem
  Logical Operator{1,4..6} (4 alike) : Logic  AllPortsSameDT=off  OutDataTypeStr=boolean
  Logical Operator2 : Logic  Operator=NOT  AllPortsSameDT=off  OutDataTypeStr=boolean
  Logical Operator3 : Logic  Operator=OR  AllPortsSameDT=off  OutDataTypeStr=boolean
  OR : Logic  Operator=OR  AllPortsSameDT=off  OutDataTypeStr=boolean
  P_Gain : Constant  Value=single(40)
  Product : Product
  Product1 : Product
  Product2 : Product
  Relational Operator : RelationalOperator  Operator=<  OutDataTypeStr=boolean  RndMeth=Simplest
  Relational Operator1 : RelationalOperator  Operator=<  OutDataTypeStr=boolean  RndMeth=Simplest
  Relational Operator2 : RelationalOperator  OutDataTypeStr=boolean  RndMeth=Simplest
  Relational Operator7 : RelationalOperator  Operator=<  OutDataTypeStr=boolean  RndMeth=Simplest
  Relational Operator8 : RelationalOperator  Operator=>  OutDataTypeStr=boolean  RndMeth=Simplest
  ResetDelay : Constant  Value=single(0.1)
  RisingTimer : Subsystem
  Saturation : Saturate  UpperLimit=40  LowerLimit=0
  Saturation Dynamic : simulink/Discontinuities/Saturation Dynamic  OutMin=[]  OutMax=[]  OutDataTypeStr=Inherit: Same as second input  OutDataType=fixdt(1, 16)  OutScaling=2^-10  DoSatur=off
  Saturation Dynamic1 : simulink/Discontinuities/Saturation Dynamic  OutMin=[]  OutMax=[]  OutDataTypeStr=Inherit: Same as second input  OutDataType=fixdt(1, 16)  OutScaling=2^-10  DoSatur=off
  Saturation Dynamic2 : simulink/Discontinuities/Saturation Dynamic  OutMin=[]  OutMax=[]  OutDataTypeStr=Inherit: Same as second input  OutDataType=fixdt(1, 16)  OutScaling=2^-10  DoSatur=off
  Saturation1 : Saturate  UpperLimit=50  LowerLimit=0
  Saturation2 : Saturate  UpperLimit=400  LowerLimit=-100
  Switch{,1..3,5..7} (7 alike) : Switch  Criteria=u2 ~= 0
  TCS_TrqRequest_Max2 : Constant  Value=single(235)
  TCS_TrqRequest_Min1 : Constant  Value=single(0)
  TCS_TrqRequest_Min2 : Constant  Value=single(0)
  Trq_IReset : Constant  Value=single(0)
  Trq_I_FF : Constant  Value=single(20)
  Unit Delay{,1..5} (6 alike) : UnitDelay  SampleTime=-1  HasFrameUpgradeWarning=on
  VehSpd_SlipTarget_mps : Lookup_n-D  NumberOfTableDimensions=1  BreakpointsForDimension1=[0,3,25,30]  Table=[0.3,0.3,2.5,2.5]  ExtrapMethod=Clip  InternalRulePriority=Speed  RndMeth=Simplest  InputSameDT=on
  VehicleStableTarget_mps : Lookup_n-D  NumberOfTableDimensions=1  BreakpointsForDimension1=[0,3,25,30]  Table=[0.4,0.4,1.2,1.2]  ExtrapMethod=Clip  InternalRulePriority=Speed  RndMeth=Simplest  InputSameDT=on
  VehicleStableTarget_mps1 : Lookup_n-D  NumberOfTableDimensions=1  BreakpointsForDimension1=[0,3,25,30]  Table=[0.4,0.4,1.2,1.2]  ExtrapMethod=Clip  InternalRulePriority=Speed  RndMeth=Simplest  InputSameDT=on
  Verror : Constant  Value=single(0)
  Verror1 : Constant  Value=single(0)
  Verror_Reset : Constant  Value=single(0)
  Verror_Reset1 : Constant  Value=single(0)
  TCSR_flgActv : Outport
  TCSR_TrqRequestFinal_Nm : Outport  Port=2
  wires:
  Add1/1 -> Unit Delay5/1, Product2/1, Switch6/1, [Verr_mps]
  Switch2/1 -> Switch5/1, Unit Delay2/1  "TCSFL_TrqRequestFinal_Nm"
  Saturation/1 -> Add9/2, VehSpd_SlipTarget_mps/1, [VehSpd_Ref_mps]
  Gain3/1 -> Saturation Dynamic/3
  [P_Portion] -> Gain3/1
  P_Gain/1 -> Product/2
  Unit Delay/1 -> Switch3/3
  Add2/1 -> Saturation2/1
  [TrqRequst_Act_Nm] -> Add11/1
  Saturation2/1 -> Unit Delay/1, Add6/1
  Switch/1 -> Add6/2  "Trq_I_Start"
  Saturation Dynamic/1 -> Add7/2  "I_Out"
  VehSpd_mps/1 -> Saturation/1  "VehSpd_mps"
  Saturation1/1 -> Add1/2, [VehSpd_RA_mps]
  Product1/1 -> Saturation Dynamic/2  "I_Portion"
  TrqRequst_Act_Nm/1 -> Add4/1, [TrqRequst_Act_Nm]
  Add6/1 -> Product1/1
  TCS_TrqRequest_Min1/1 -> Saturation Dynamic2/3
  Detect Rise Positive/1 -> Switch/2
  Integr_StartPoint/1 -> Switch/3
  I_Gain/1 -> Product1/2
  Saturation Dynamic2/1 -> Switch2/1  "TCS_TrqRequest"
  Add7/1 -> Saturation Dynamic1/2, [TCS_TrqReqstRaw_Nm]  "TCS_TrqReqst_Raw"
  [TrqRequst_Act_Nm] -> Saturation Dynamic2/2
  VehSpd_SlipTarget_mps/1 -> Add9/1
  Add9/1 -> Add1/1
  [Verr_mps] -> Relational Operator7/1
  Cal_DeltaV_mps/1 -> Relational Operator7/2
  Relational Operator7/1 -> Latch_on/1(Set), Logical Operator2/1  "TCS_Trigger"
  [TCS_TrqReqstRaw_Nm] -> Unit Delay4/1
  Logical Operator2/1 -> Logical Operator1/1
  Relational Operator8/1 -> Logical Operator1/2  "fSat_Actuators"
  Cal_DeltaV_mps1/1 -> Relational Operator8/2
  Logical Operator1/1 -> RisingTimer/1(Set)
  ResetDelay/1 -> RisingTimer/2(Timer)
  RisingTimer/1(TCSExit) -> Logical Operator3/1
  Logical Operator3/1 -> Latch_on/2(Reset)  "TCS_ExitFinal"
  Latch_on/1(flg_TCSActv) -> TCSR_flgActv/1, [TCS_Actv]
  [TCS_Actv] -> Switch6/2
  Verror_Reset/1 -> Switch6/3
  Switch6/1 -> Product/1, Add2/2  "Verror_mps"
  Product/1 -> [P_Portion], Add7/1  "P_out"
  [TCS_Actv] -> Detect Rise Positive/1
  [P_Portion] -> Unit Delay1/1
  Add4/1 -> Switch/1
  Unit Delay1/1 -> Add4/2
  [VehSpd_Ref_mps] -> Add5/1, VehicleStableTarget_mps/1
  VehicleStableTarget_mps/1 -> Add5/2
  Add5/1 -> Add10/2
  [VehSpd_RA_mps] -> Add10/1
  Add10/1 -> Relational Operator/1
  Verror/1 -> Relational Operator/2
  Relational Operator/1 -> Logical Operator4/1
  [TCS_Actv] -> Logical Operator4/2
  Logical Operator4/1 -> Switch1/2  "flg_I_FF"
  Trq_I_FF/1 -> Switch1/1
  Trq_IReset/1 -> Switch1/3
  Switch1/1 -> Add6/3  "Trq_I_FF"
  [P_Portion] -> Add11/2
  Add11/1 -> Saturation Dynamic/1
  [TCS_Actv] -> Switch2/2
  Switch7/1 -> Switch2/3
  [TrqRequst_Act_Nm] -> Switch7/1
  Verror1/1 -> Relational Operator1/2
  Add12/1 -> Relational Operator1/1
  [VehSpd_RA_mps] -> Add12/1
  Add13/1 -> Add12/2
  VehicleStableTarget_mps1/1 -> Add13/2
  [VehSpd_Ref_mps] -> VehicleStableTarget_mps1/1, Add13/1
  [TCS_TrqReqstRaw_Nm] -> Compare To Constant2/1, Relational Operator2/1
  [TrqRequst_Act_Nm] -> Relational Operator2/2
  Relational Operator1/1 -> Logical Operator5/1
  Relational Operator2/1 -> OR/1
  Logical Operator5/1 -> Unit Delay3/1, Switch7/2  "TCS_Inactive"
  Unit Delay3/1 -> [TCS_Inactive]
  [TCS_Inactive] -> Logical Operator3/2
  Unit Delay4/1 -> Relational Operator8/1
  VehSpdFL_mps/1 -> Saturation1/1  "VehSpdFL_mps"
  Saturation Dynamic1/1 -> Saturation Dynamic2/1
  TCS_TrqRequest_Max2/1 -> Saturation Dynamic1/1
  TCS_TrqRequest_Min2/1 -> Saturation Dynamic1/3
  Switch3/1 -> Add2/1
  Verror_Reset1/1 -> Switch3/1
  [Verr_Zore] -> Switch3/2
  Unit Delay5/1 -> Product2/2
  Product2/1 -> Compare To Constant/1
  Compare To Constant/1 -> [Verr_Zore]
  <StrWhlAng>/1 -> Abs/1
  Compare To Zero/1 -> Logical Operator6/1
  Abs/1 -> Compare To Constant1/1
  [VehSpd_RA_mps] -> Compare To Zero/1
  Compare To Constant1/1 -> Logical Operator6/2
  Unit Delay2/1 -> Switch7/3
  Switch5/1 -> TCSR_TrqRequestFinal_Nm/1
  Logical Operator6/1 -> Switch5/2
  [TrqRequst_Act_Nm] -> Switch5/3
  Compare To Constant2/1 -> OR/2
  OR/1 -> Logical Operator5/2

== system VehCtrlMdel240829_2018b/Input/ABS_Receive/ABS_BUS_state ==
  CANOK : Inport
  ID : Inport  Port=2
  Msg : Inport  Port=3
  function : TriggerPort  TriggerType=function-call  VariantControl=(inherit)
  Bus Creator3 : BusCreator  Inputs=4
  IMU_state : Subsystem  TreatAsAtomicUnit=on
  ABS_BUS : Outport  VectorParamsAs1DForOutWhenUnconnected=off
  wires:
  IMU_state/3(ABS_WS_FL) -> Bus Creator3/3
  IMU_state/2(ABS_WS_RL) -> Bus Creator3/2
  IMU_state/1(ABS_WS_FR) -> Bus Creator3/1
  Bus Creator3/1 -> ABS_BUS/1
  ID/1 -> IMU_state/1(ID)
  CANOK/1 -> IMU_state/Enable
  Msg/1 -> IMU_state/2(Msg)
  IMU_state/4(ABS_WS_RR) -> Bus Creator3/4

== system VehCtrlMdel240829_2018b/Input/AMKMCU_Receive/FLAMKMCU ==
  AMKMCU_state : Subsystem  TreatAsAtomicUnit=on
  AMKMCU_state1 : Subsystem  TreatAsAtomicUnit=on
  AMKMCU_state2 : Subsystem  TreatAsAtomicUnit=on
  CANReceive1 : ec5744lib/RapidECU_U3/04CANCommunication/CANReceive  canmodule=1  canbuffer=2  canmessageid=642  canmessagetype=Standard(11-bit ID)  datalength=8  sampletime=-1
      settings: SourceProductName=ECUCoder for MPC5744
  CANReceive2 : ec5744lib/RapidECU_U3/04CANCommunication/CANReceive  canmodule=1  canbuffer=3  canmessageid=644  canmessagetype=Standard(11-bit ID)  datalength=8  sampletime=-1
      settings: SourceProductName=ECUCoder for MPC5744
  CANReceive3 : ec5744lib/RapidECU_U3/04CANCommunication/CANReceive  canmodule=1  canbuffer=1  canmessageid=640  canmessagetype=Standard(11-bit ID)  datalength=8  sampletime=-1
      settings: SourceProductName=ECUCoder for MPC5744
  Terminator1 : Terminator
  Terminator2 : Terminator
  Terminator3 : Terminator
  FLAMKMCUtoVCU1 : Outport  VectorParamsAs1DForOutWhenUnconnected=off
  FLAMKMCUtoVCU2 : Outport  Port=2  VectorParamsAs1DForOutWhenUnconnected=off
  FLAMKMCUtoVCU3 : Outport  Port=3  VectorParamsAs1DForOutWhenUnconnected=off
  wires:
  CANReceive2/2 -> AMKMCU_state2/1(CANOK)
  CANReceive1/4 -> AMKMCU_state1/3(Msg)
  CANReceive3/5 -> Terminator3/1
  CANReceive1/3 -> AMKMCU_state1/2(ID)
  CANReceive1/1 -> AMKMCU_state1/Trigger
  CANReceive2/4 -> AMKMCU_state2/3(Msg)
  CANReceive3/3 -> AMKMCU_state/2(ID)
  CANReceive3/2 -> AMKMCU_state/1(CANOK)
  CANReceive2/3 -> AMKMCU_state2/2(ID)
  CANReceive1/2 -> AMKMCU_state1/1(CANOK)
  CANReceive1/5 -> Terminator1/1
  CANReceive3/4 -> AMKMCU_state/3(Msg)
  CANReceive2/5 -> Terminator2/1
  CANReceive3/1 -> AMKMCU_state/Trigger
  CANReceive2/1 -> AMKMCU_state2/Trigger
  AMKMCU_state2/1(FLAMKMCUtoVCU3) -> FLAMKMCUtoVCU3/1  "FLAMKMCUtoVCU3"
  AMKMCU_state/1(FLAMKtoVCU1) -> FLAMKMCUtoVCU1/1
  AMKMCU_state1/1(FLAMKMCUtoVCU2) -> FLAMKMCUtoVCU2/1  "FLAMKMCUtoVCU2"

== system VehCtrlMdel240829_2018b/Input/AMKMCU_Receive/FRAMKMCU ==
  AMKMCU_state : Subsystem  TreatAsAtomicUnit=on
  AMKMCU_state1 : Subsystem  TreatAsAtomicUnit=on
  AMKMCU_state2 : Subsystem  TreatAsAtomicUnit=on
  CANReceive1 : ec5744lib/RapidECU_U3/04CANCommunication/CANReceive  canmodule=1  canbuffer=5  canmessageid=643  canmessagetype=Standard(11-bit ID)  datalength=8  sampletime=-1
      settings: SourceProductName=ECUCoder for MPC5744
  CANReceive2 : ec5744lib/RapidECU_U3/04CANCommunication/CANReceive  canmodule=1  canbuffer=6  canmessageid=387  canmessagetype=Standard(11-bit ID)  datalength=8  sampletime=-1
      settings: SourceProductName=ECUCoder for MPC5744
  CANReceive3 : ec5744lib/RapidECU_U3/04CANCommunication/CANReceive  canmodule=1  canbuffer=4  canmessageid=641  canmessagetype=Standard(11-bit ID)  datalength=8  sampletime=-1
      settings: SourceProductName=ECUCoder for MPC5744
  Terminator1 : Terminator
  Terminator2 : Terminator
  Terminator3 : Terminator
  FRAMKMCUtoVCU1 : Outport  VectorParamsAs1DForOutWhenUnconnected=off
  FRAMKMCUtoVCU2 : Outport  Port=2  VectorParamsAs1DForOutWhenUnconnected=off
  FRAMKMCUtoVCU3 : Outport  Port=3  VectorParamsAs1DForOutWhenUnconnected=off
  wires:
  AMKMCU_state1/1(FRAMKMCUtoVCU2) -> FRAMKMCUtoVCU2/1  "FRAMKMCUtoVCU2"
  AMKMCU_state/1(FRAMKMCUtoVCU1) -> FRAMKMCUtoVCU1/1  "FRAMKMCUtoVCU1"
  AMKMCU_state2/1(FRAMKMCUtoVCU3) -> FRAMKMCUtoVCU3/1  "FRAMKMCUtoVCU3"
  CANReceive2/1 -> AMKMCU_state2/Trigger
  CANReceive3/1 -> AMKMCU_state/Trigger
  CANReceive2/5 -> Terminator2/1
  CANReceive3/4 -> AMKMCU_state/3(Msg)
  CANReceive1/5 -> Terminator1/1
  CANReceive1/2 -> AMKMCU_state1/1(CANOK)
  CANReceive2/3 -> AMKMCU_state2/2(ID)
  CANReceive3/2 -> AMKMCU_state/1(CANOK)
  CANReceive3/3 -> AMKMCU_state/2(ID)
  CANReceive2/4 -> AMKMCU_state2/3(Msg)
  CANReceive1/1 -> AMKMCU_state1/Trigger
  CANReceive1/3 -> AMKMCU_state1/2(ID)
  CANReceive3/5 -> Terminator3/1
  CANReceive1/4 -> AMKMCU_state1/3(Msg)
  CANReceive2/2 -> AMKMCU_state2/1(CANOK)

== system VehCtrlMdel240829_2018b/Input/BMS_Recive/ABS_BUS_state ==
  CANOK : Inport
  ID : Inport  Port=2
  Msg : Inport  Port=3
  function : TriggerPort  TriggerType=function-call  VariantControl=(inherit)
  Bus Creator : BusCreator  Inputs=9
  IMU_state : Subsystem  TreatAsAtomicUnit=on
  BMS_BUS : Outport  VectorParamsAs1DForOutWhenUnconnected=off
  wires:
  Bus Creator/1 -> BMS_BUS/1
  ID/1 -> IMU_state/1(ID)
  CANOK/1 -> IMU_state/Enable
  Msg/1 -> IMU_state/2(Msg)
  IMU_state/1(BatAlmlv) -> Bus Creator/1
  IMU_state/2(BatLife) -> Bus Creator/2
  IMU_state/3(BatState) -> Bus Creator/3
  IMU_state/4(LSBAz) -> Bus Creator/4
  IMU_state/5(LSBVz) -> Bus Creator/5
  IMU_state/6(MSBAz) -> Bus Creator/6
  IMU_state/7(MSBVz) -> Bus Creator/7
  IMU_state/8(SOCz) -> Bus Creator/8
  IMU_state/9(SOHz) -> Bus Creator/9

== system VehCtrlMdel240829_2018b/Input/EMRAXMCU_RECIEVE/MCU_pwr ==
  CANOK : Inport
  ID : Inport  Port=2
  Msg : Inport  Port=3
  function : TriggerPort  TriggerType=function-call  VariantControl=(inherit)
  Bus Creator3 : BusCreator  Inputs=5
  MCU_VCUMeter1 : Subsystem  TreatAsAtomicUnit=on
  MCU_pwr : Outport
  wires:
  Bus Creator3/1 -> MCU_pwr/1
  Msg/1 -> MCU_VCUMeter1/2(Msg)
  CANOK/1 -> MCU_VCUMeter1/Enable
  ID/1 -> MCU_VCUMeter1/1(ID)
  MCU_VCUMeter1/1("AC_current ") -> Bus Creator3/1  "AC_current"
  MCU_VCUMeter1/2(MCU_temp) -> Bus Creator3/2  "MCU_temp"
  MCU_VCUMeter1/3(current) -> Bus Creator3/3  "current"
  MCU_VCUMeter1/4(motor_temp) -> Bus Creator3/4  "motor_temp"
  MCU_VCUMeter1/5(voltage) -> Bus Creator3/5  "voltage"

== system VehCtrlMdel240829_2018b/Input/EMRAXMCU_RECIEVE/MCU_state ==
  CANOK : Inport
  ID : Inport  Port=2
  Msg : Inport  Port=3
  function : TriggerPort  TriggerType=function-call  VariantControl=(inherit)
  Bus Creator3 : BusCreator  Inputs=15
  MCU_state : Subsystem  TreatAsAtomicUnit=on
  Out1 : Outport  VectorParamsAs1DForOutWhenUnconnected=off
  wires:
  Msg/1 -> MCU_state/2(Msg)
  CANOK/1 -> MCU_state/Enable
  ID/1 -> MCU_state/1(ID)
  Bus Creator3/1 -> Out1/1
  MCU_state/1(12V_error) -> Bus Creator3/1
  MCU_state/2(alarm) -> Bus Creator3/2
  MCU_state/3(undervol) -> Bus Creator3/3
  MCU_state/4(controller_ready) -> Bus Creator3/4
  MCU_state/5(MCU_temp_warn) -> Bus Creator3/5
  MCU_state/6(mode_cmd8) -> Bus Creator3/6
  MCU_state/7(motor_temp_warn) -> Bus Creator3/7
  MCU_state/8(overcur) -> Bus Creator3/8
  MCU_state/9(pow_lim_warn) -> Bus Creator3/9
  MCU_state/10(overvol) -> Bus Creator3/10
  MCU_state/11(precharge) -> Bus Creator3/11
  MCU_state/12(rotation_warn) -> Bus Creator3/12
  MCU_state/13(selfcech) -> Bus Creator3/13
  MCU_state/14(RPM) -> Bus Creator3/14
  MCU_state/15(torque) -> Bus Creator3/15
